simulink model "dq0inverter_refined_meow"  (R2023b)
settings: Solver=VariableStepAuto  StartTime=0.0  StopTime=30
libraries: spsCurrentMeasurementLib x6, spsSeriesRLCBranchLib x5, spsIGBTDiodeLib x4, simulink x3, dspstat3 x3, spsBreakerLib x2, slpidlib x2, spsPWMGenerator2LevelLib x2, spsSeriesRLCLoadLib x2, spsdq0toabcLib x2, spsVoltageMeasurementLib x2, spsACVoltageSourceLib x1
settings Model: Creator=Jia Yee Wong  LastModifiedBy=Jia Yee Wong
settings HardwareCC: ProdBitPerLong=64  ProdLargestAtomicFloat=None  ProdHWDeviceType=AMD->Athlon 64
settings SFSimCC: SimUserIncludeDirs=C:\JJ\FinalYearProject  SimTargetLang=C++
settings SFSimCC: SimCustomHeaderCode=|
  | #include "referencegen.h"
  | #include "zerocrossingenable.h"
settings SFSimCC: SimUserSources=|
  | referencegen.cpp;
  | zerocrossingenable.c;

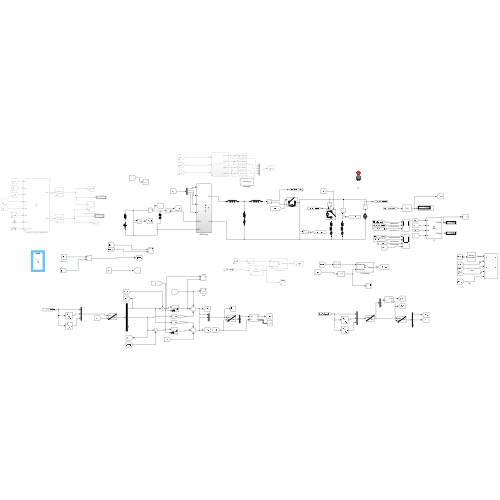
[thumbnail: Simulink's stored preview of the top-level diagram]
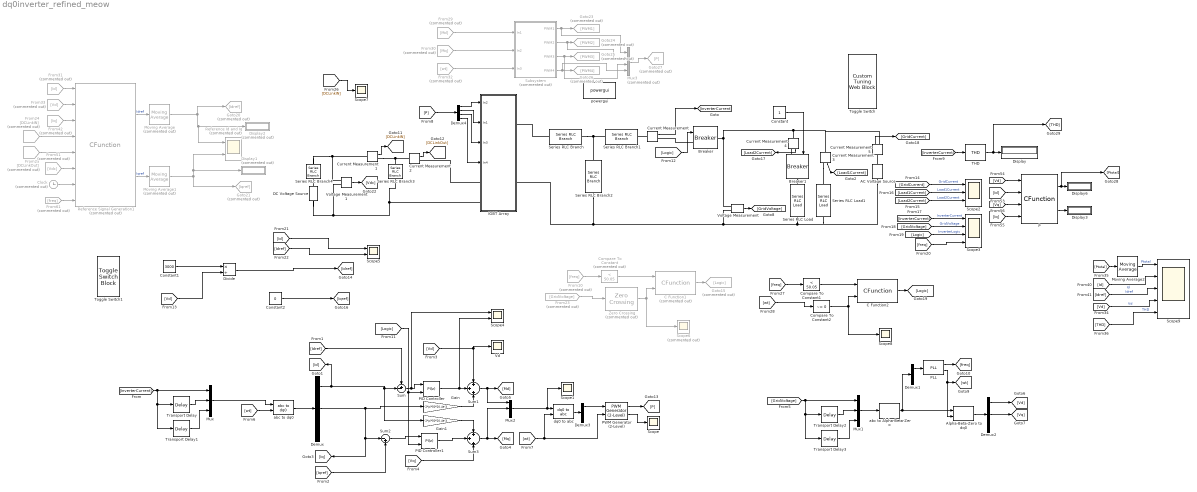
== system dq0inverter_refined_meow ==
  AC Voltage Source : spsACVoltageSourceLib/AC Voltage Source  Amplitude=340  Phase=0  Frequency=50  SampleTime=0  Measurements=Voltage  BusType=PQ  Pref=3000  Qref=0  Qmin=-inf  Qmax=+inf
  Alpha-Beta-Zero to dq0 : spsAlphaBetaZerotodq0Lib/Alpha-Beta-Zero to dq0  Alignment=90 degrees behind phase A axis
  Breaker : spsBreakerLib/Breaker  InitialState=0  SwitchingTimes="[1/60  5/60]"  External=on  BreakerResistance=0.01  SnubberResistance=1e6  SnubberCapacitance=47e-3  Measurements=None  MoreParameters=on  NoBreakLoop=off
  Breaker1 : spsBreakerLib/Breaker  InitialState=0  SwitchingTimes="[1/60  5/60]"  External=on  BreakerResistance=0.01  SnubberResistance=1e6  SnubberCapacitance=inf  Measurements=None  MoreParameters=on  NoBreakLoop=off
  C Function1 : CFunction  Commented=on  OutputCode=|  SampleTime=1/50000
      | if(Frequency == true && ZeroCross==1){
      |     Output = 1;}
      | else if(Frequency == false){
      |         Output = 0;}
  C Function2 : CFunction  OutputCode=|  SampleTime=1/50000
      | if(Frequency == true && ZeroCross==1){
      |     Output = 1;}
      | else if(Frequency == false){
      |         Output = 0;}
  Clock : Clock  Commented=on
  Compare To Constant : simulink/Logic and Bit Operations/Compare To Constant  Commented=on  relop=<  const=50.05  OutDataTypeStr=boolean
  Compare To Constant1 : simulink/Logic and Bit Operations/Compare To Constant  relop=<  const=50.05  OutDataTypeStr=boolean
  Compare To Constant2 : simulink/Logic and Bit Operations/Compare To Constant  relop=~=  const=0  OutDataTypeStr=boolean
  Constant : Constant
  Constant1 : Constant  Value=3000
  Constant2 : Constant  Value=0
  Current Measurement{,1..5} (6 alike) : spsCurrentMeasurementLib/Current Measurement  PhasorSimulation=off  OutputType=Complex  PSBequivalent=0
  DC Voltage Source : spsDCVoltageSourceLib/DC Voltage Source  Amplitude=400  Measurements=None
  Demux{,1..3} (4 alike) : Demux  Outputs=3
  Demux4 : Demux
  Display : Display
  Display1 : Display  Commented=on
  Display2 : Display  Commented=on
  Display3 : Display
  Display6 : Display
  Divide : Product  Inputs=*/
  From10 : From  Commented=on  GotoTag=freq
  From23 : From  Commented=on  GotoTag=GridVoltage
  From24 : From  Commented=on  GotoTag=DCLinkIN
  From25 : From  Commented=on  GotoTag=DCLinkOut
  From29 : From  Commented=on  GotoTag=Md
  From30 : From  Commented=on  GotoTag=Mq
  From31 : From  Commented=on  GotoTag=Id
  From32 : From  Commented=on  GotoTag=wt
  From33 : From  Commented=on  GotoTag=Vd
  From42 : From  Commented=on  GotoTag=Iq
  From51 : From  Commented=on  GotoTag=Vdc
  From61 : From  Commented=on  GotoTag=freq
  Gain : Gain  Gain=-2*pi*50*20.4e-3
  Gain1 : Gain  Gain=-2*pi*50*20.4e-3
  Goto15 : Goto  Commented=on  GotoTag=Logic
  Goto20 : Goto  Commented=on  GotoTag=Idref
  Goto21 : Goto  Commented=on  GotoTag=Iqref
  Goto23 : Goto  Commented=on  GotoTag=PWM1
  Goto24 : Goto  Commented=on  GotoTag=PWM2
  Goto25 : Goto  Commented=on  GotoTag=PWM3
  Goto26 : Goto  Commented=on  GotoTag=PWM4
  Goto27 : Goto  Commented=on  GotoTag=P
  IGBT Array : Subsystem
  Moving Average : dspstat3/Moving Average  Commented=on  Method=Sliding window  ForgettingFactorPort=off  SpecifyWindowLength=on  WindowLength=4  OverlapLength=3  AllowArbitraryInputLength=off  ForgettingFactor=0.9  SimulateUsing=Code generation
  Moving Average1 : dspstat3/Moving Average  Commented=on  Method=Sliding window  ForgettingFactorPort=off  SpecifyWindowLength=on  WindowLength=4  OverlapLength=3  AllowArbitraryInputLength=off  ForgettingFactor=0.9  SimulateUsing=Code generation
  Moving Average2 : dspstat3/Moving Average  Method=Sliding window  ForgettingFactorPort=off  SpecifyWindowLength=on  WindowLength=4  OverlapLength=3  AllowArbitraryInputLength=off  ForgettingFactor=0.9  SimulateUsing=Code generation
  Mux : Mux  Inputs=3
  Mux1 : Mux  Inputs=3
  Mux2 : Mux  Inputs=3
  Mux3 : Mux  Commented=on
  P : CFunction  OutputCode=|
      | PTotal = Id*Vd;
      | QTotal = Vq*Id;
  PID Controller : slpidlib/PID Controller  Controller=PI  Form=Parallel  TimeDomain=Discrete-time  UseExternalTs=off  SampleTime=1/50000  IntegratorMethod=Forward Euler  FilterMethod=Forward Euler  ControllerParametersSource=internal  P=30  I=20  UseKiTs=off  D=0  N=100  UseFilter=on  TunerSelectOption=Transfer Function Based (PID Tuner App)  ZeroCross=off  InitialConditionSource=internal  InitialConditionForIntegrator=0  InitialConditionForFilter=0  DifferentiatorICPrevScaledInput=0  ExternalReset=either  TrackingMode=off  Kt=1  LimitOutput=on  SatLimitsSource=internal  UpperSaturationLimit=30  LowerSaturationLimit=-1000  LinearizeAsGain=on  AntiWindupMode=back-calculation  Kb=1  LimitIntegrator=on  UpperIntegratorSaturationLimit=30  LowerIntegratorSaturationLimit=-1000  POutMin=[]  POutMax=[]  IOutMin=[]  IOutMax=[]  DOutMin=[]  DOutMax=[]  NOutMin=[]  NOutMax=[]  SumOutMin=[]  SumOutMax=[]  SaturationOutMin=[]  SaturationOutMax=[]  PParamMin=[]  PParamMax=[]  IParamMin=[]  IParamMax=[]  DParamMin=[]  DParamMax=[]  NParamMin=[]  NParamMax=[]  KbParamMin=[]  KbParamMax=[]  KtParamMin=[]  KtParamMax=[]  KbOutMin=[]  KbOutMax=[]  KtOutMin=[]  KtOutMax=[]  IntegratorOutMin=[]  IntegratorOutMax=[]  FilterOutMin=[]  FilterOutMax=[]  SumI1OutMin=[]  SumI1OutMax=[]  SumI2OutMin=[]  SumI2OutMax=[]  SumI3OutMin=[]  SumI3OutMax=[]  SumI4OutMin=[]  SumI4OutMax=[]  SumDOutMin=[]  SumDOutMax=[]  DifferentiatorOutMin=[]  DifferentiatorOutMax=[]  FilterDiffOutCoefMin=[]  FilterDiffOutCoefMax=[]  ReciprocalOutMin=[]  ReciprocalOutMax=[]  SumDenOutMin=[]  SumDenOutMax=[]  SumNumOutMin=[]  SumNumOutMax=[]  DivideOutMin=[]  DivideOutMax=[]  UdiffTsProdOutMin=[]  UdiffTsProdOutMax=[]  NTsProdOutMin=[]  NTsProdOutMax=[]  UintegralTsProdOutMin=[]  UintegralTsProdOutMax=[]  UngainTsProdOutMin=[]  UngainTsProdOutMax=[]  ClampingZeroOutDataTypeStr=Inherit: Inherit via back propagation  ClampingZeroOutMin=[]  ClampingZeroOutMax=[]  FilterDenConstantOutDataTypeStr=Inherit: Inherit via back propagation  FilterDenConstantOutMin=[]  FilterDenConstantOutMax=[]  PCopyOutDataTypeStr=Inherit: Inherit via back propagation  PCopyOutMin=[]  PCopyOutMax=[]  NCopyOutDataTypeStr=Inherit: Inherit via back propagation  NCopyOutMin=[]  NCopyOutMax=[]  IntegratorContinuousStateAttributes=''  IntegratorStateMustResolveToSignalObject=off  IntegratorRTWStateStorageClass=Auto  FilterContinuousStateAttributes=''  FilterStateMustResolveToSignalObject=off  FilterRTWStateStorageClass=Auto  ParallelPVariant=InternalParameters  IdealPVariant=Disabled  IVariant=InternalParameters  DVariant=Disabled  IntegratorVariant=Discrete  SatVariant=Enabled  AWVariant=BackCalculation  PCopyVariant=Disabled  TRVariant=Disabled  FdbkBlocksVariant=Forward  IdealPFdbkVariant=Disabled  SatFdbkVariant=Disabled  DerivativeFilterVariant=Disabled  NVariant=Disabled  NCopyVariant=Disabled_SignalSpec  FilterICVariant=Disabled  IntegratorICVariant=InternalICs  ExternalResetVariant=ExternalReset  TRSumVariant=Passthrough  SumFdbkVariant=Disabled  SumVariant=Sum_PI  TsampFilterVariant=InternalTs  TsampNgainVariant=Passthrough  TsampIntegralVariant=Disabled_SignalSpec  ExternalSaturationOutDataTypeStr=Inherit: Same as second input
  PID Controller1 : slpidlib/PID Controller  Controller=PI  Form=Parallel  TimeDomain=Discrete-time  UseExternalTs=off  SampleTime=1/50000  IntegratorMethod=Forward Euler  FilterMethod=Forward Euler  ControllerParametersSource=internal  P=30  I=20  UseKiTs=off  D=0  N=100  UseFilter=on  TunerSelectOption=Transfer Function Based (PID Tuner App)  InitialConditionSource=internal  InitialConditionForIntegrator=0  InitialConditionForFilter=0  DifferentiatorICPrevScaledInput=0  ExternalReset=either  TrackingMode=off  Kt=1  LimitOutput=on  SatLimitsSource=internal  UpperSaturationLimit=30  LowerSaturationLimit=-1000  LinearizeAsGain=on  AntiWindupMode=back-calculation  Kb=1  LimitIntegrator=on  UpperIntegratorSaturationLimit=30  LowerIntegratorSaturationLimit=-1000  POutMin=[]  POutMax=[]  IOutMin=[]  IOutMax=[]  DOutMin=[]  DOutMax=[]  NOutMin=[]  NOutMax=[]  SumOutMin=[]  SumOutMax=[]  SaturationOutMin=[]  SaturationOutMax=[]  PParamMin=[]  PParamMax=[]  IParamMin=[]  IParamMax=[]  DParamMin=[]  DParamMax=[]  NParamMin=[]  NParamMax=[]  KbParamMin=[]  KbParamMax=[]  KtParamMin=[]  KtParamMax=[]  KbOutMin=[]  KbOutMax=[]  KtOutMin=[]  KtOutMax=[]  IntegratorOutMin=[]  IntegratorOutMax=[]  FilterOutMin=[]  FilterOutMax=[]  SumI1OutMin=[]  SumI1OutMax=[]  SumI2OutMin=[]  SumI2OutMax=[]  SumI3OutMin=[]  SumI3OutMax=[]  SumI4OutMin=[]  SumI4OutMax=[]  SumDOutMin=[]  SumDOutMax=[]  DifferentiatorOutMin=[]  DifferentiatorOutMax=[]  FilterDiffOutCoefMin=[]  FilterDiffOutCoefMax=[]  ReciprocalOutMin=[]  ReciprocalOutMax=[]  SumDenOutMin=[]  SumDenOutMax=[]  SumNumOutMin=[]  SumNumOutMax=[]  DivideOutMin=[]  DivideOutMax=[]  UdiffTsProdOutMin=[]  UdiffTsProdOutMax=[]  NTsProdOutMin=[]  NTsProdOutMax=[]  UintegralTsProdOutMin=[]  UintegralTsProdOutMax=[]  UngainTsProdOutMin=[]  UngainTsProdOutMax=[]  ClampingZeroOutDataTypeStr=Inherit: Inherit via back propagation  ClampingZeroOutMin=[]  ClampingZeroOutMax=[]  FilterDenConstantOutDataTypeStr=Inherit: Inherit via back propagation  FilterDenConstantOutMin=[]  FilterDenConstantOutMax=[]  PCopyOutDataTypeStr=Inherit: Inherit via back propagation  PCopyOutMin=[]  PCopyOutMax=[]  NCopyOutDataTypeStr=Inherit: Inherit via back propagation  NCopyOutMin=[]  NCopyOutMax=[]  IntegratorContinuousStateAttributes=''  IntegratorStateMustResolveToSignalObject=off  IntegratorRTWStateStorageClass=Auto  FilterContinuousStateAttributes=''  FilterStateMustResolveToSignalObject=off  FilterRTWStateStorageClass=Auto  ParallelPVariant=InternalParameters  IdealPVariant=Disabled  IVariant=InternalParameters  DVariant=Disabled  IntegratorVariant=Discrete  SatVariant=Enabled  AWVariant=BackCalculation  PCopyVariant=Disabled  TRVariant=Disabled  FdbkBlocksVariant=Forward  IdealPFdbkVariant=Disabled  SatFdbkVariant=Disabled  DerivativeFilterVariant=Disabled  NVariant=Disabled  NCopyVariant=Disabled_SignalSpec  FilterICVariant=Disabled  IntegratorICVariant=InternalICs  ExternalResetVariant=ExternalReset  TRSumVariant=Passthrough  SumFdbkVariant=Disabled  SumVariant=Sum_PI  TsampFilterVariant=InternalTs  TsampNgainVariant=Passthrough  TsampIntegralVariant=Disabled_SignalSpec  ExternalSaturationOutDataTypeStr=Inherit: Same as second input
  PLL : spsPLLLib/PLL  Fmin=49.95  Par_Init=[0, 51]  ParK=[180, 3200, 1]  TcD=1e-4  MaxRateChangeFreq=12  FilterCutOffFreq=25  Ts=0  AGC=on
      settings: LibrarySourceBlock=sps_lib/Control/PLL
  PWM Generator (2-Level) : spsPWMGenerator2LevelLib/PWM Generator (2-Level)  ModulatorType=Single-phase full-bridge - Bipolar modulation (4 pulses)  ModulatorMode=Synchronized  Fc=27*60  Pc=90  nF=200  MinMax="[ -10  10 ]"  SamplingTechnique=Natural  ModulatingSignals=off  m=0.8  Freq=60  Phase=0  Ts=1/5000  ShowCarrierOutport=on
  Reference Id and Iq : Scope  Commented=on  NumInputPorts=2
  Reference Signal Generation1 : CFunction  Commented=on  OutputCode=|  StartCode=|  SampleTime=1/50000
      OutputCode=|
      | if(Id!=PreviousId || Iq!=PreviousIq){
      |     if(ReferenceGenTrigger(Freq_PLL)){
      |         Idref_buffer=IdrefCalc(CLK,Vd,Iin,Iout, Vdc, Vdc);
      |         if(Idref_buffer<0){
      |             Idref=-Idref_buffer;}
      |         else if(Idref_buffer >9){
      |                Idref=9;} 
      |         else {Idref=Idref_buffer;}
      |   //Idref =3000/Vd;
      |    Iqref=-1;
      |    PreviousId=Id;
      |    PreviousIq=Iq;
      |    }
      |   
      | } else { Idref = 0; Iqref = 0;}
      StartCode=|
      | PreviousIq =0;
      | PreviousId =0;
  Scope{,1,7..8} (4 alike) : Scope
  Scope2 : Scope  NumInputPorts=3
  Scope3 : Scope  NumInputPorts=4
  Scope4 : Scope  NumInputPorts=2
  Scope5 : Scope  NumInputPorts=2
  Scope6 : Scope  Commented=on
  Scope9 : Scope  NumInputPorts=5
  Series RLC Branch : spsSeriesRLCBranchLib/Series RLC Branch  LConnTagsString=__new0  RConnTagsString=__new0  BranchType=L  Resistance=0.1  Inductance=20.4e-3  SetiL0=off  InitialCurrent=0  Capacitance=1e-6  Setx0=off  InitialVoltage=0  Measurements=None
  Series RLC Branch1 : spsSeriesRLCBranchLib/Series RLC Branch  LConnTagsString=__new0  RConnTagsString=__new0  BranchType=L  Resistance=0.1  Inductance=148e-6  SetiL0=off  InitialCurrent=0  Capacitance=1e-6  Setx0=off  InitialVoltage=0  Measurements=None
  Series RLC Branch2 : spsSeriesRLCBranchLib/Series RLC Branch  LConnTagsString=__new0  RConnTagsString=__new0  BranchType=RC  Resistance=100  Inductance=1e-3  SetiL0=off  InitialCurrent=0  Capacitance=5.6e-6  Setx0=off  InitialVoltage=0  Measurements=None
  Series RLC Branch3 : spsSeriesRLCBranchLib/Series RLC Branch  LConnTagsString=__new0  RConnTagsString=__new0  BranchType=RC  Resistance=1  Inductance=1e-3  SetiL0=off  InitialCurrent=0  Capacitance=100e-3  Setx0=off  InitialVoltage=0  Measurements=None
  Series RLC Branch4 : spsSeriesRLCBranchLib/Series RLC Branch  LConnTagsString=__new0  RConnTagsString=__new0  BranchType=R  Resistance=10  Inductance=1e-3  SetiL0=off  InitialCurrent=0  Capacitance=47e-3  Setx0=off  InitialVoltage=0  Measurements=None
  Series RLC Load : spsSeriesRLCLoadLib/Series RLC Load  LConnTagsString=a  RConnTagsString=__new0  NominalVoltage=240  NominalFrequency=50  ActivePower=5e3  InductivePower=200  CapacitivePower=100  Setx0=off  InitialVoltage=0  SetiL0=off  InitialCurrent=0  Measurements=Branch voltage and current  LoadType=constant PQ
  Series RLC Load1 : spsSeriesRLCLoadLib/Series RLC Load  LConnTagsString=a  RConnTagsString=__new0  NominalVoltage=240  NominalFrequency=50  ActivePower=6e3  InductivePower=100  CapacitivePower=100  Setx0=off  InitialVoltage=0  SetiL0=off  InitialCurrent=0  Measurements=None  LoadType=constant PQ
  Subsystem : Subsystem  Commented=on
  Sum : Sum  Inputs=+-|
  Sum1 : Sum  Inputs=+|+|+
  Sum2 : Sum  Inputs=|-+
  Sum3 : Sum  Inputs=+|+|+
  THD : spsTHDLib/THD  Freq=50  Ts=1/50000
  Toggle Switch : CustomTuningWebBlock  LabelPosition=Hide  ShowInitialText=on  Configuration="{\"components\":[{\"name\":\"CustomSwitchStateComponent\",\"settings\":{\"position\":[0,0,1,1],\"showAllLabels\":1,\"states\":[{\"HitRegion\":{\"position\":[0.5,0,1,0.5]},\"Image\":{\"position\":[0,0.24928571428571428,0.5014285714285714,1],\"size\":[0.5014285714285714,1],\"src\":\"data:image\\/svg+xml;base64,PHN2ZyB4bWxucz0iaHR0cDovL3d3dy53My5vcmcvMjAwMC9zdmciIHhtbG5zOnhsaW5rPSJodHRwOi8vd3d3LnczLm9yZy8xOTk5L3hsaW5rIiB2aWV3Qm94PSIwIDAgMzguMDQgMTUwIj48ZGVmcz48c3R5bGU+LmNscy0xe2ZpbGw6dXJsKCNyYWRpYWwtZ3JhZGllbnQpO30uY2xzLTJ7ZmlsbDp1cmwoI3JhZGlhbC1ncmFkaWVudC0yKTt9LmNscy0ze2ZpbGw6dXJsKCNXaGl0ZV9CbGFjayk7fS5jbHMtNHtmaWxsOnVybCgjcmFkaWFsLWdyYWRpZW50LTMpO30uY2xzLTV7ZmlsbDojNWI1YjViO30uY2xzLTZ7ZmlsbDp1cmwoI3Jh ...(+3556 chars)\",\"srcOrientation\":\"Right\"},\"Label\":{\"color\":[0.5019607843137255,0.5019607843137255,0.5019607843137255],\"icon\":{\"size\":[0,0],\"src\":[],\"srcOrientation\":\"Right\"},\"iconPlacement\":\"left\",\"opacity\":1,\"position\":[0.92,0.5],\"show\":true,\"text\":{\"content\":\"Off\",\"font\":\"Helvetica\",\"fontSize\":24.5}},\"Value\":0},{\"HitRegion\":{\"position\":[0,0,1,0.5]},\"Image\":{\"position\":[0,0.24928571428571428,0.5014285714285714,1],\"size\":[0.5014285714285714,1],\"src\":\"data:image\\/svg+xml;base64,PHN2ZyB4bWxucz0iaHR0cDovL3d3dy53My5vcmcvMjAwMC9zdmciIHhtbG5zOnhsaW5rPSJodHRwOi8vd3d3LnczLm9yZy8xOTk5L3hsaW5rIiB2aWV3Qm94PSIwIDAgMzguMDQgMTUwIj48ZGVmcz48c3R5bGU+LmNscy0xe2ZpbGw6dXJsKCNyYWRpYWwtZ3JhZGllbnQpO30uY2xzLTJ7ZmlsbDp1cmwoI3JhZGlhbC1ncmFkaWVudC0yKTt9LmNscy0ze2ZpbGw6dXJsKCNXaGl0ZV9CbGFjayk7fS5jbHMtNHtmaWxsOnVybCgjcmFkaWFsLWdyYWRpZW50LTMpO30uY2xzLTV7ZmlsbDojNWI1YjViO30uY2xzLTZ7ZmlsbDp1cmwoI3Jh ...(+3628 chars)\",\"srcOrientation\":\"Right\"},\"Label\":{\"color\":[0.5019607843137255,0.5019607843137255,0.5019607843137255],\"icon\":{\"size\":[0,0],\"src\":[],\"srcOrientation\":\"Right\"},\"iconPlacement\":\"left\",\"opacity\":1,\"position\":[0.08,0.5],\"show\":true,\"text\":{\"content\":\"On\",\"font\":\"Helvetica\",\"fontSize\":24.5}},\"Value\":1}]}},{\"name\":\"BackgroundImageComponent\",\"settings\":{\"image\":{\"size\":[70,135],\"src\":\"default\",\"srcOrientation\":\"Right\"},\"position\":[0,0,1,1],\"scaleMode\":\"0\"}},{\"name\":\"ForegroundImageComponent\",\"settings\":{\"image\":{\"size\":[0,0],\"src\":\"default\",\"srcOrientation\":[]},\"isForeground\":1,\"position\":[0,0,1,1],\"scaleMode\":\"0\"}}],\"settings\":{\"BindingType\":\"param\",\"backgroundColor\":[0,0,0],\"backgroundOffset\":0.14,\"fixedAspectRatio\":\"on\",\"foregroundColor\":[0,0,0],\"showBackgroundColor\":false,\"variant\":\"toggle\",\"version\":\"R2023a\"},\"type\":\"Switch\"}"
  Toggle Switch1 : ToggleSwitchBlock
      settings: Values={{'Off', 'On'}, [2000 3000]}
  Transport Delay : TransportDelay  DelayTime=6.67e-3  BufferSize=4096
  Transport Delay1 : TransportDelay  DelayTime=13.34e-3  BufferSize=4096
  Transport Delay2 : TransportDelay  DelayTime=6.67e-3  BufferSize=4096  FixedBuffer=on  TransDelayFeedthrough=on
  Transport Delay3 : TransportDelay  DelayTime=13.34e-3  BufferSize=4096  FixedBuffer=on  TransDelayFeedthrough=on
  Vd : Scope
  Voltage Measurement : spsVoltageMeasurementLib/Voltage Measurement  PhasorSimulation=off  OutputType=Complex  PSBequivalent=0
  Voltage Measurement1 : spsVoltageMeasurementLib/Voltage Measurement  PhasorSimulation=off  OutputType=Complex  PSBequivalent=0
  Zero Crossing : dspsigops/Zero Crossing  Commented=on  InputProcessing=Columns as channels (frame based)
  abc to Alpha-Beta-Zero : spsabctoAlphaBetaZeroLib/abc to Alpha-Beta-Zero
  abc to dq0 : spsabctodq0Lib/abc to dq0  Alignment=Aligned with phase A axis
  dq0 to abc : spsdq0toabcLib/dq0 to abc  Alignment=Aligned with phase A axis
  powergui : sps_lib/powergui  Priority=1  SimulationMode=Continuous  SampleTime=50e-6  frequency=50  Iterations=50  frequencyindice=50  Pbase=100e6  ErrMax=1e-4  UnitsV=kV  UnitsW=MW  buscounter=0  FunctionMessages=off  echomessages=off  EnableUseOfTLC=off  CurrentSourceSwitches=off  DisableSnubberDevices=off  DisableRonSwitches=off  DisableVfSwitches=off  DisplayEquations=off  AutomaticDiscreteSolvers=off  SolverType=Backward Euler  Interpol=off  ExternalGateDelay=off  methode=off  Ts=100  x0status=zero  SPID=on  SwTol=0  HookPort=off  NonlinearTolerance=1e-4  nMaxIteration=100  ContinueOnMaxIteration=off  RestoreLinks=warning  ResistiveCurrentMeasurement=off  Frange=[0:2:500]  Ylog=off  Xlog=on  ShowGrid=off  save=off  variable=ZData  structure=0  ZoomFFT=off  StartTime=0.0  cycles=1  DisplayStyle=1  fundamental=60  FreqAxis=off  MaxFrequency=1000  frequencyindicesteady=1  RmsSteady=1  display=off
  wires:
  Current Measurement/1 -> [InverterCurrent]
  Transport Delay/1 -> Mux/2
  [InverterCurrent] -> Transport Delay1/1, Transport Delay/1, Mux/1
  Transport Delay1/1 -> Mux/3
  Demux/1 -> [Id], Gain1/1, Sum/2
  [Idref] -> Sum/1
  PID Controller/1 -> Scope4/2, Sum1/2
  Demux/2 -> [Iq], Sum2/1, Gain/1
  Gain/1 -> Sum1/3
  Sum1/1 -> Mux2/1, [Md]
  Sum3/1 -> Mux2/2, [Mq]
  Transport Delay3/1 -> Mux1/3
  Mux1/1 -> abc to Alpha-Beta-Zero/1
  [GridVoltage] -> Transport Delay3/1, Transport Delay2/1, Mux1/1
  Transport Delay2/1 -> Mux1/2
  abc to Alpha-Beta-Zero/1 -> Demux1/1, Alpha-Beta-Zero to dq0/1
  Demux1/1 -> PLL/1
  PLL/2 -> [wt], Alpha-Beta-Zero to dq0/2
  Alpha-Beta-Zero to dq0/1 -> Demux2/1
  Demux2/2 -> [Vq]
  Demux2/1 -> [Vd]
  Voltage Measurement/1 -> [GridVoltage]
  PLL/1 -> [freq]
  [wt] -> abc to dq0/2
  Current Measurement1/1 -> [DCLinkIN]
  Current Measurement2/1 -> [DCLinkOut]
  dq0 to abc/1 -> Demux3/1
  [wt] -> dq0 to abc/2, PWM Generator (2-Level)/2
  Demux3/1 -> PWM Generator (2-Level)/1
  PWM Generator (2-Level)/1 -> [P]
  From10/1 -> Compare To Constant/1
  [InverterCurrent] -> THD/1
  THD/1 -> [THD], Display/1
  PWM Generator (2-Level)/2 -> Scope/1
  Constant/1 -> Breaker1/1
  Current Measurement3/1 -> [Load1Current]
  Current Measurement4/1 -> [Load2Current]
  Current Measurement5/1 -> [GridCurrent]
  [Load1Current] -> Scope2/2  "Load1Current"
  [Load2Current] -> Scope2/3  "Load2Current"
  [GridCurrent] -> Scope2/1  "GridCurrent"
  [InverterCurrent] -> Scope3/1  "InverterCurrent"
  [GridVoltage] -> Scope3/2  "GridVoltage"
  [Logic] -> Scope3/3  "InverterLogic"
  [freq] -> Scope3/4
  [Id] -> Scope5/1
  Mux2/1 -> Scope1/1, dq0 to abc/1
  Constant2/1 -> [Iqref]
  abc to dq0/1 -> Demux/1
  Gain1/1 -> Sum3/1
  [Iqref] -> Sum2/2
  Mux/1 -> abc to dq0/1
  Demux4/1 -> IGBT Array/1(In2)
  Demux4/2 -> IGBT Array/2(In1)
  Demux4/3 -> IGBT Array/3(In3)
  Demux4/4 -> IGBT Array/4(In4)
  [P] -> Demux4/1
  [Logic] -> Breaker/1
  PID Controller1/1 -> Sum3/2
  Sum2/1 -> PID Controller1/1
  Sum/1 -> Scope4/1, PID Controller/1
  [Vd] -> Sum1/1, Vd/1
  [Vq] -> Sum3/3
  [Logic] -> PID Controller1/2, PID Controller/2
  Divide/1 -> [Idref]
  Constant1/1 -> Divide/1
  [Vd] -> Divide/2
  [Idref] -> Scope5/2
  C Function1/1 -> Goto15/1
  Compare To Constant/1 -> C Function1/1
  From23/1 -> Zero Crossing/1
  Zero Crossing/1 -> C Function1/2, Scope6/1
  From25/1 -> Reference Signal Generation1/5
  Clock/1 -> Reference Signal Generation1/7
  From61/1 -> Reference Signal Generation1/8
  From33/1 -> Reference Signal Generation1/2
  From24/1 -> Reference Signal Generation1/4
  From51/1 -> Reference Signal Generation1/6
  From42/1 -> Reference Signal Generation1/3
  From31/1 -> Reference Signal Generation1/1
  Voltage Measurement1/1 -> [Vdc]
  Reference Signal Generation1/2 -> Moving Average1/1  "Iqref"
  Reference Signal Generation1/1 -> Moving Average/1  "Idref"
  Moving Average/1 -> Reference Id and Iq/1, Display2/1, Goto20/1
  Moving Average1/1 -> Display1/1, Reference Id and Iq/2, Goto21/1
  [Id] -> P/2
  P/2 -> Display3/1
  [Vd] -> P/1
  [Iq] -> P/4
  [Vq] -> P/3
  P/1 -> [Ptotal], Display6/1
  [DCLinkIN] -> Scope7/1
  C Function2/1 -> [Logic]
  Compare To Constant1/1 -> C Function2/1
  Compare To Constant2/1 -> C Function2/2, Scope8/1
  [freq] -> Compare To Constant1/1
  [wt] -> Compare To Constant2/1
  From32/1 -> Subsystem/3(In3)
  Subsystem/2(PWM2) -> Mux3/2, Goto24/1
  From29/1 -> Subsystem/1(In1)
  Subsystem/4(PWM4) -> Mux3/4, Goto26/1
  From30/1 -> Subsystem/2(In2)
  Subsystem/1(PWM1) -> Mux3/1, Goto23/1
  Subsystem/3(PWM3) -> Mux3/3, Goto25/1
  Mux3/1 -> Goto27/1
  [Vd] -> Scope9/4  "Vd"
  [Ptotal] -> Moving Average2/1
  Moving Average2/1 -> Scope9/1  "Ptotal"
  [Id] -> Scope9/2  "Id"
  [Idref] -> Scope9/3  "Idref"
  [THD] -> Scope9/5  "THD"
  connections:
  Series RLC Branch/RConn1 -- Series RLC Branch2/LConn1 -- Series RLC Branch1/LConn1
  Breaker/RConn1 -- Current Measurement5/RConn1 -- Current Measurement3/LConn1 -- Current Measurement4/LConn1 -- Voltage Measurement/LConn1
  Series RLC Branch2/RConn1 -- IGBT Array/RConn2 -- Series RLC Load1/RConn1 -- AC Voltage Source/LConn1 -- Series RLC Load/RConn1 -- Voltage Measurement/LConn2
  Current Measurement/LConn1 -- Series RLC Branch1/RConn1
  Breaker/LConn1 -- Current Measurement/RConn1
  Series RLC Branch/LConn1 -- IGBT Array/RConn1
  Current Measurement1/RConn1 -- Current Measurement2/LConn1 -- Series RLC Branch3/LConn1
  DC Voltage Source/RConn1 -- Series RLC Branch4/RConn1
  DC Voltage Source/LConn1 -- Voltage Measurement1/LConn2 -- IGBT Array/LConn2 -- Series RLC Branch3/RConn1
  Series RLC Load/LConn1 -- Breaker1/RConn1
  Current Measurement3/RConn1 -- Series RLC Load1/LConn1
  Current Measurement4/RConn1 -- Breaker1/LConn1
  AC Voltage Source/RConn1 -- Current Measurement5/LConn1
  Series RLC Branch4/LConn1 -- Voltage Measurement1/LConn1 -- Current Measurement1/LConn1
  IGBT Array/LConn1 -- Current Measurement2/RConn1

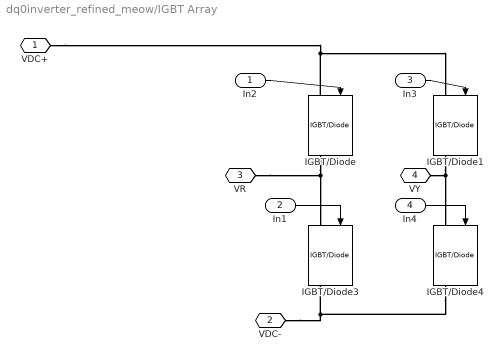
== system dq0inverter_refined_meow/IGBT Array ==
  In2 : Inport
  In1 : Inport  Port=2
  In3 : Inport  Port=3
  In4 : Inport  Port=4
  IGBT/Diode{,1,3..4} (4 alike) : spsIGBTDiodeLib/IGBT//Diode  Ron=1e-3  Rs=1e5  Cs=inf  Measurements=on
  VDC+ : PMIOPort  Side=Left
  VDC- : PMIOPort  Port=2  Side=Left
  VR : PMIOPort  Port=3  Side=Right
  VY : PMIOPort  Port=4  Side=Right
  wires:
  In1/1 -> IGBT/Diode3/1
  In4/1 -> IGBT/Diode4/1
  In3/1 -> IGBT/Diode1/1
  In2/1 -> IGBT/Diode/1
  connections:
  IGBT/Diode4/RConn1 -- VDC-/RConn1 -- IGBT/Diode3/RConn1
  IGBT/Diode/RConn1 -- VR/RConn1 -- IGBT/Diode3/LConn1
  IGBT/Diode1/RConn1 -- VY/RConn1 -- IGBT/Diode4/LConn1
  IGBT/Diode/LConn1 -- VDC+/RConn1 -- IGBT/Diode1/LConn1

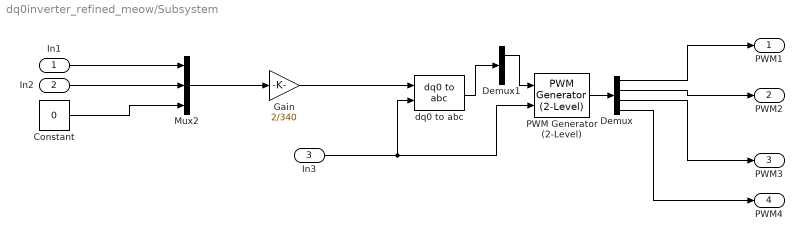
== system dq0inverter_refined_meow/Subsystem ==
  In1 : Inport
  In2 : Inport  Port=2
  In3 : Inport  Port=3
  Constant : Constant  Value=0
  Demux : Demux
  Demux1 : Demux  Outputs=3
  Gain : Gain  Gain=2/340
  Mux2 : Mux  Inputs=3
  PWM Generator (2-Level) : spsPWMGenerator2LevelLib/PWM Generator (2-Level)  ModulatorType=Single-phase full-bridge (4 pulses)  ModulatorMode=Synchronized  Fc=27*60  Pc=90  nF=27  MinMax="[ -1  1 ]"  SamplingTechnique=Natural  ModulatingSignals=off  m=0.8  Freq=60  Phase=0  Ts=1/50000  ShowCarrierOutport=off
  dq0 to abc : spsdq0toabcLib/dq0 to abc  Alignment=90 degrees behind phase A axis
  PWM1 : Outport
  PWM2 : Outport  Port=2
  PWM3 : Outport  Port=3
  PWM4 : Outport  Port=4
  wires:
  Mux2/1 -> Gain/1
  In1/1 -> Mux2/1
  In2/1 -> Mux2/2
  In3/1 -> PWM Generator (2-Level)/2, dq0 to abc/2
  PWM Generator (2-Level)/1 -> Demux/1
  Demux/1 -> PWM1/1
  Demux/2 -> PWM2/1
  Demux/3 -> PWM3/1
  Demux/4 -> PWM4/1
  Constant/1 -> Mux2/3
  dq0 to abc/1 -> Demux1/1
  Demux1/1 -> PWM Generator (2-Level)/1
  Gain/1 -> dq0 to abc/1
